simulink model "multi_kanal_V2"  (R2024a)
settings: Solver=VariableStepAuto  StartTime=0.0  StopTime=1000  RelTol=1e-9  AbsTol=1e-10
libraries: simulink x13, matrix_library x3, sharedutil x2, aerolibutil x1
settings Model: Creator=evgenijkondratev  LastModifiedBy=evgenijkondratev

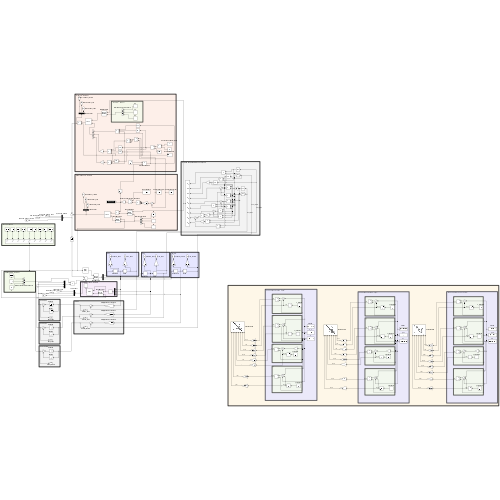
[thumbnail: Simulink's stored preview of the top-level diagram]
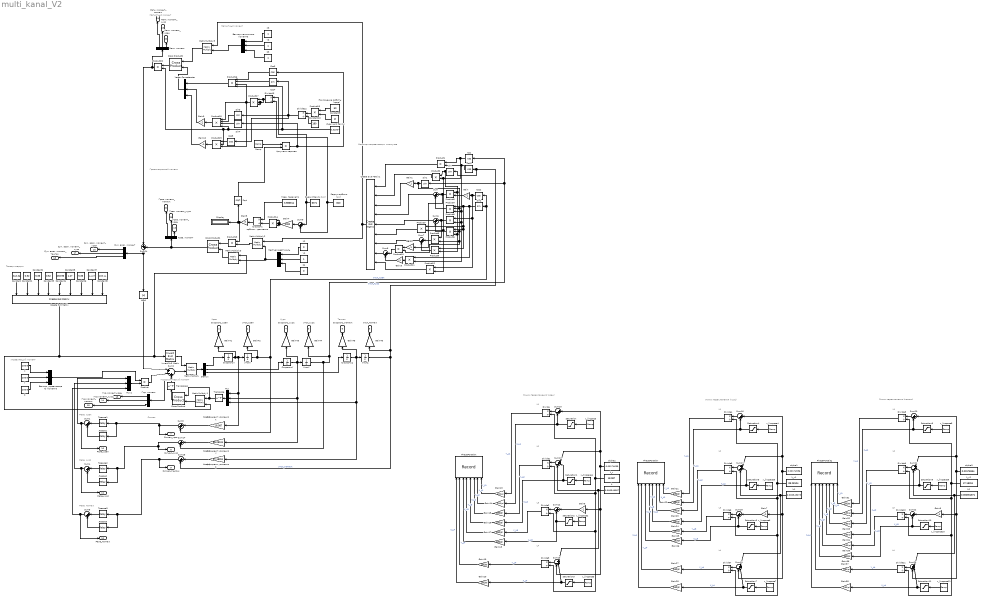
== system multi_kanal_V2 ==
  note: L3
  note: L4
  note: Крен
  note: Магнитный момент
  note: Линии переключения (крен)
  note: L4
  note: Линии переключения (курс)
  note: Линии переключения (тангаж)
  note: L3
  note: L1
  note: Реле, тангаж
  note: L2
  note: L4
  note: L1
  note: L1
  note: L3
  note: Сигнал
  note: Матрица направляющих косинусов
  note: Тензор инерции
  note: L2
  note: Реле, курс
  note: L2
  note: Управляющий момент
  note: Курс
  note: Тангаж
  note: Реле, крен
  note: Гироскопический момент
  note: Гравитационный момент
  note: Магнитный момент
  Abs1 : Abs  SaturateOnIntegerOverflow=off
  Constant : Constant  Value=363.86
  Constant1 : Constant  Value=0.52
  Constant10 : Constant  Value=180
  Constant2 : Constant  Value=5.36
  Constant3 : Constant  Value=0.52
  Constant4 : Constant  Value=233.96
  Constant5 : Constant  Value=1.27
  Constant6 : Constant  Value=5.36
  Constant7 : Constant  Value=14.27
  Constant8 : Constant  Value=285.14
  Constant9 : Constant  Value=pi
  Cos{,1..3,5} (5 alike) : Trigonometry  Operator=cos
  Cos4 : Trigonometry
  Create 3x3 Matrix : sharedutil/Create 3x3 Matrix  aMode=aMode
      settings: LibrarySourceBlock=aerolibutil/Create 3x3 Matrix
  Create 3x3 Matrix1 : sharedutil/Create 3x3 Matrix  aMode=aMode
      settings: LibrarySourceBlock=aerolibutil/Create 3x3 Matrix
  Cross Product : matrix_library/Cross Product
  Cross Product1 : matrix_library/Cross Product
  Cross Product2 : matrix_library/Cross Product
  Demux : Demux  Outputs=3
  Display : Display
  Divide{,1..13} (14 alike) : Product  Inputs=*/
  Gain{,1..3,6..8,10} (8 alike) : Gain  Gain=-1
  Gain{13..28,31..38,41..46} (30 alike) : Gain  Gain=180/pi
  Gain4 : Gain  Gain=1000
  Gain5 : Gain  Gain=3
  Gain9 : Gain  Gain=-2
  Invert 3x3 Matrix : aerolibutil/Invert  3x3 Matrix
  MatrixMultiply{,1..3,5} (5 alike) : Product  Multiplication=Matrix(*)
  Mux : Mux  Inputs=3
  Mux1 : Mux  Inputs=3
  PhasePortraitX : Record  FileSettingsInternal="{\"entries\":[{\"content\":{\"excelSettings\":{\"content\":{},\"type\":\"Streamout.ExcelSettings\"}},\"type\":\"Streamout.FileSettingStorage\",\"uuid\":\"\"}],\"packageUris\":[\"http:\\/\\/schema.mathworks.com\\/mf0\\/streamout_blocks\\/R2020a\"],\"version\":\"1.0\"}"  Layout=[1 1]  SignalsInternal="{\"entries\":[{\"content\":{\"signals\":[{\"content\":{\"blockPath\":[],\"dimensions\":[1],\"domain\":\"\",\"lineColor\":\"#7e2f8e\",\"lineWidth\":2,\"port\":1,\"sid\":[\"\"],\"signalID\":1,\"signalName\":\"X_L4\"},\"type\":\"RecordBlkView.Signal\",\"uuid\":\"\"},{\"content\":{\"blockPath\":[],\"dimensions\":[1],\"domain\":\"\",\"lineColor\":\"#77ac30\",\"lineWidth\":2,\"port\":2,\"sid\":[\"\"],\"signalID\":2,\"signalName\":\"Y_L4\"},\"type\":\"RecordBlkView.Signal\",\"uuid\":\"\"},{\"content\":{\"blockPath\":[],\"dimensions\":[1],\"domain\":\"\",\"lineColor\":\"#4dbeee\",\"lineWidth\":2,\"port\":3,\"sid\":[\"\"],\"signalID\":3,\"signalName\":\"X_L3\"},\"type\":\"RecordBlkView.Signal\",\"uuid\":\"\"},{\"content\":{\"blockPath\":[],\"dimensions\":[1],\"domain\":\"\",\"lineColor\":\"#a2142f\",\"lineWidth\":2,\"port\":4,\"sid\":[\"\"],\"signalID\":4,\"signalName\":\"Y_L3\"},\"type\":\"RecordBlkView.Signal\",\"uuid\":\"\"},{\"content\":{\"blockPath\":[],\"dimensions\":[1],\"domain\":\"\",\"lineColor\":\"#139fff\",\"lineWidth\":2,\"port\":5,\"sid\":[\"\"],\"signalID\":5,\"signalName\":\"X_L2\"},\"type\":\"RecordBlkView.Signal\",\"uuid\":\"\"},{\"content\":{\"blockPath\":[],\"dimensions\":[1],\"domain\":\"\",\"lineColor\":\"#ff6929\",\"lineWidth\":2,\"port\":6,\"sid\":[\"\"],\"signalID\":6,\"signalName\":\"Y_L2\"},\"type\":\"RecordBlkView.Signal\",\"uuid\":\"\"},{\"content\":{\"blockPath\":[],\"dimensions\":[1],\"domain\":\"\",\"lineColor\":\"#b746ff\",\"lineWidth\":2,\"port\":7,\"sid\":[\"\"],\"signalID\":7,\"signalName\":\"X_L1\"},\"type\":\"RecordBlkView.Signal\",\"uuid\":\"\"},{\"content\":{\"blockPath\":[],\"dimensions\":[1],\"domain\":\"\",\"lineColor\":\"#64d413\",\"lineWidth\":2,\"port\":8,\"sid\":[\"\"],\"signalID\":8,\"signalName\":\"Y_L1\"},\"type\":\"RecordBlkView.Signal\",\"uuid\":\"\"}]},\"type\":\"RecordBlkView.InputSignals\",\"uuid\":\"\"}],\"packageUris\":[\"http:\\/\\/schema.mathworks.com\\/mf0\\/streamout_blocks\\/R2020a\"],\"version\":\"1.0\"}"  VisualizationBindings="{\"xyplotplugin\":{\"info\":[{\"series\":[],\"subplotID\":1}]}}"  CompatibilityTag=XY
  PhasePortraitY : Record  FileSettingsInternal="{\"entries\":[{\"content\":{\"excelSettings\":{\"content\":{},\"type\":\"Streamout.ExcelSettings\"}},\"type\":\"Streamout.FileSettingStorage\",\"uuid\":\"\"}],\"packageUris\":[\"http:\\/\\/schema.mathworks.com\\/mf0\\/streamout_blocks\\/R2020a\"],\"version\":\"1.0\"}"  Layout=[1 1]  SignalsInternal="{\"entries\":[{\"content\":{\"signals\":[{\"content\":{\"blockPath\":[],\"dimensions\":[1],\"domain\":\"\",\"lineColor\":\"#4dbeee\",\"lineWidth\":2,\"port\":1,\"sid\":[\"\"],\"signalID\":1,\"signalName\":\"X_L4\"},\"type\":\"RecordBlkView.Signal\",\"uuid\":\"\"},{\"content\":{\"blockPath\":[],\"dimensions\":[1],\"domain\":\"\",\"lineColor\":\"#a2142f\",\"lineWidth\":2,\"port\":2,\"sid\":[\"\"],\"signalID\":2,\"signalName\":\"Y_L4\"},\"type\":\"RecordBlkView.Signal\",\"uuid\":\"\"},{\"content\":{\"blockPath\":[],\"dimensions\":[1],\"domain\":\"\",\"lineColor\":\"#139fff\",\"lineWidth\":2,\"port\":3,\"sid\":[\"\"],\"signalID\":3,\"signalName\":\"X_L3\"},\"type\":\"RecordBlkView.Signal\",\"uuid\":\"\"},{\"content\":{\"blockPath\":[],\"dimensions\":[1],\"domain\":\"\",\"lineColor\":\"#ff6929\",\"lineWidth\":2,\"port\":4,\"sid\":[\"\"],\"signalID\":4,\"signalName\":\"Y_L3\"},\"type\":\"RecordBlkView.Signal\",\"uuid\":\"\"},{\"content\":{\"blockPath\":[],\"dimensions\":[1],\"domain\":\"\",\"lineColor\":\"#b746ff\",\"lineWidth\":2,\"port\":5,\"sid\":[\"\"],\"signalID\":5,\"signalName\":\"X_L2\"},\"type\":\"RecordBlkView.Signal\",\"uuid\":\"\"},{\"content\":{\"blockPath\":[],\"dimensions\":[1],\"domain\":\"\",\"lineColor\":\"#64d413\",\"lineWidth\":2,\"port\":6,\"sid\":[\"\"],\"signalID\":6,\"signalName\":\"Y_L2\"},\"type\":\"RecordBlkView.Signal\",\"uuid\":\"\"},{\"content\":{\"blockPath\":[],\"dimensions\":[1],\"domain\":\"\",\"lineColor\":\"#ff13a6\",\"lineWidth\":2,\"port\":7,\"sid\":[\"\"],\"signalID\":7,\"signalName\":\"X_L1\"},\"type\":\"RecordBlkView.Signal\",\"uuid\":\"\"},{\"content\":{\"blockPath\":[],\"dimensions\":[1],\"domain\":\"\",\"lineColor\":\"#fe330a\",\"lineWidth\":2,\"port\":8,\"sid\":[\"\"],\"signalID\":8,\"signalName\":\"Y_L1\"},\"type\":\"RecordBlkView.Signal\",\"uuid\":\"\"}]},\"type\":\"RecordBlkView.InputSignals\",\"uuid\":\"\"}],\"packageUris\":[\"http:\\/\\/schema.mathworks.com\\/mf0\\/streamout_blocks\\/R2020a\"],\"version\":\"1.0\"}"  VisualizationBindings="{\"xyplotplugin\":{\"info\":[{\"series\":[],\"subplotID\":1}]}}"  CompatibilityTag=XY
  PhasePortraitZ : Record  FileSettingsInternal="{\"entries\":[{\"content\":{\"excelSettings\":{\"content\":{},\"type\":\"Streamout.ExcelSettings\"}},\"type\":\"Streamout.FileSettingStorage\",\"uuid\":\"\"}],\"packageUris\":[\"http:\\/\\/schema.mathworks.com\\/mf0\\/streamout_blocks\\/R2020a\"],\"version\":\"1.0\"}"  Layout=[1 1]  SignalsInternal="{\"entries\":[{\"content\":{\"signals\":[{\"content\":{\"blockPath\":[],\"dimensions\":[1],\"domain\":\"\",\"lineColor\":\"#22b573\",\"lineWidth\":2,\"plots\":[ 1 ],\"port\":1,\"sid\":[\"\"],\"signalID\":1,\"signalName\":\"X_L4\"},\"type\":\"RecordBlkView.Signal\",\"uuid\":\"\"},{\"content\":{\"blockPath\":[],\"dimensions\":[1],\"domain\":\"\",\"lineColor\":\"#7e2f8e\",\"lineWidth\":2,\"plots\":[ 1 ],\"port\":2,\"sid\":[\"\"],\"signalID\":2,\"signalName\":\"Y_L4\"},\"type\":\"RecordBlkView.Signal\",\"uuid\":\"\"},{\"content\":{\"blockPath\":[],\"dimensions\":[1],\"domain\":\"\",\"lineColor\":\"#fe330a\",\"lineWidth\":2,\"port\":3,\"sid\":[\"\"],\"signalID\":3,\"signalName\":\"X_L3\"},\"type\":\"RecordBlkView.Signal\",\"uuid\":\"\"},{\"content\":{\"blockPath\":[],\"dimensions\":[1],\"domain\":\"\",\"lineColor\":\"#22b573\",\"lineWidth\":2,\"port\":4,\"sid\":[\"\"],\"signalID\":4,\"signalName\":\"Y_L3\"},\"type\":\"RecordBlkView.Signal\",\"uuid\":\"\"},{\"content\":{\"blockPath\":[],\"dimensions\":[1],\"domain\":\"\",\"lineColor\":\"#0072bd\",\"lineWidth\":2,\"port\":5,\"sid\":[\"\"],\"signalID\":5,\"signalName\":\"X_L2\"},\"type\":\"RecordBlkView.Signal\",\"uuid\":\"\"},{\"content\":{\"blockPath\":[],\"dimensions\":[1],\"domain\":\"\",\"lineColor\":\"#64d413\",\"lineWidth\":2,\"port\":6,\"sid\":[\"\"],\"signalID\":6,\"signalName\":\"Y_L2\"},\"type\":\"RecordBlkView.Signal\",\"uuid\":\"\"},{\"content\":{\"blockPath\":[],\"dimensions\":[1],\"domain\":\"\",\"lineColor\":\"#edb120\",\"lineWidth\":2,\"port\":7,\"sid\":[\"\"],\"signalID\":7,\"signalName\":\"X_L1\"},\"type\":\"RecordBlkView.Signal\",\"uuid\":\"\"},{\"content\":{\"blockPath\":[],\"dimensions\":[1],\"domain\":\"\",\"lineColor\":\"#7e2f8e\",\"lineWidth\":2,\"port\":8,\"sid\":[\"\"],\"signalID\":8,\"signalName\":\"Y_L1\"},\"type\":\"RecordBlkView.Signal\",\"uuid\":\"\"}]},\"type\":\"RecordBlkView.InputSignals\",\"uuid\":\"\"}],\"packageUris\":[\"http:\\/\\/schema.mathworks.com\\/mf0\\/streamout_blocks\\/R2020a\"],\"version\":\"1.0\"}"  VisualizationBindings="{\"xyplotplugin\":{\"info\":[{\"series\":[{\"bindingParametersList\":[{\"parameter\":\"X-Axis\",\"signalID\":1,\"signalName\":\"X_L4\"},{\"parameter\":\"Y-Axis\",\"signalID\":2,\"signalName\":\"Y_L4\"}],\"seriesID\":0}],\"subplotID\":1}]}}"  CompatibilityTag=XY
  Product{,1..3,5,7..13,15,20} (14 alike) : Product
  Product{4,6,14,17,19} (5 alike) : Product  Inputs=3
  Product16 : Product  Inputs=4
  Product18 : Product  Inputs=4
  Ramp : simulink/Sources/Ramp  slope=1  start=0  InitialOutput=0
  Saturation{,1..11} (12 alike) : Saturate  UpperLimit=0.15  LowerLimit=-0.15
  Sin{,1..4} (5 alike) : Trigonometry
  Sqrt : Sqrt
  Sum{,1,3..9,14..15,24} (12 alike) : Sum  Inputs=|++
  Sum{10,12,16,18,20,22} (6 alike) : Sum  Inputs=|+-
  Sum{11,13,17,19,21,23} (6 alike) : Sum  Inputs=|+--
  Sum2 : Sum  Inputs=|+-+
  Transpose : Math  Operator=transpose
  Transpose1 : Math  Operator=transpose
  Vector Concatenate : Concatenate  NumInputs=3
  X : Constant  Value=20e-3
  X2 : Constant  Value=0
  X3 : Constant
  Y : Constant  Value=20e-3
  Y2 : Constant
  Y3 : Constant
  Z : Constant  Value=20e-3
  Z2 : Constant  Value=0
  Z3 : Constant
  alpha1 : Constant  Value=0.00174536
  alpha2 : Constant  Value=0.00174639
  alpha3 : Constant  Value=0.00175934
  h : Constant  Value=0.000349087
  h1 : Constant  Value=0.000349073
  h2 : Constant  Value=0.000351871
  k_x : Constant  Value=18.087
  k_x1 : Constant  Value=89.28104
  k_x2 : Constant  Value=37.18251
  x_linspace{,1..11} (12 alike) : simulink/Sources/Ramp  slope=1  start=0  InitialOutput=-1
  Аргумент перигея : Product
  Вектор магнитного момента : Concatenate  NumInputs=3
  Вектор управляющего момента : Concatenate  NumInputs=3
  Гир. момент : Demux  Outputs=3
  Грав. момент : Demux  Outputs=3
  Грав. параметр : Constant  Value=3.986e14
  Индукция Земли : Constant  Value=0.315e-4
  Коэффициент усиления X : Gain  Gain=18.087
  Коэффициент усиления Y : Gain  Gain=89.28104
  Коэффициент усиления Z : Gain  Gain=37.18251
  Левое1 : Relay  OnSwitchValue=-0.00174639+0.000349087  OffSwitchValue=-0.00174639  OnOutputValue=0  OffOutputValue=-1
  Левое2 : Relay  OnSwitchValue=-0.00174536+0.000349073  OffSwitchValue=-0.00174536  OnOutputValue=0  OffOutputValue=-1
  Левое3 : Relay  OnSwitchValue=-0.00175934+0.000351871  OffSwitchValue=-0.00175934  OnOutputValue=0  OffOutputValue=-1
  Магн. момент : Demux  Outputs=3
  Местная вертикаль : Concatenate  NumInputs=3
  Наклонение орбиты (град) : Constant  Value=50
  Правое1 : Relay  OnSwitchValue=0.00174639  OffSwitchValue=0.00174639-0.000349087
  Правое2 : Relay  OnSwitchValue=0.00174536  OffSwitchValue=0.00174536-0.000349073
  Правое3 : Relay  OnSwitchValue=0.00175934  OffSwitchValue=0.00175934-0.000351871
  Радиус Земли (км) : Constant  Value=6371
  Радиус орбиты (км) : Constant  Value=820
  Скорость орбитального движения : Product  Inputs=*/
  СкоростьX : Integrator  InitialCondition=0.00053*pi/180
  СкоростьY : Integrator  InitialCondition=0.00008*pi/180
  СкоростьZ : Integrator  InitialCondition=0.00028*pi/180
  Сум. возм. момент : Demux  Outputs=3
  УголX : Integrator
  УголY : Integrator
  УголZ : Integrator
  Угол_крен : Outport
  Скорость_крен : Outport  Port=2
  Угол_курс : Outport  Port=3
  Скорость_курс : Outport  Port=4
  Угол_тангаж : Outport  Port=5
  Скорость_тангаж : Outport  Port=6
  Сигнал_крен : Outport  Port=7
  Сигнал_курс : Outport  Port=8
  Сигнал_тангаж : Outport  Port=9
  Реле_крен : Outport  Port=10
  Реле_курс : Outport  Port=11
  Реле_тангаж : Outport  Port=12
  Гир.момент_крен : Outport  Port=13
  Гир.момент_курс : Outport  Port=14
  Гир.момент_тангаж : Outport  Port=15
  Сум. возм. момент_крен : Outport  Port=16
  Сум. возм. момент_курс : Outport  Port=17
  Сум. возм. момент_тангаж : Outport  Port=18
  Грав. момент_крен : Outport  Port=19
  Грав. момент_курс : Outport  Port=20
  Грав. момент_тангаж : Outport  Port=21
  Магн. момент_крен : Outport  Port=22
  Магн. момент_курс : Outport  Port=23
  Магн. момент_тангаж : Outport  Port=24
  wires:
  Y2/1 -> Местная вертикаль/2
  Sum17/1 -> Divide5/1
  Ramp/1 -> Аргумент перигея/1
  Z/1 -> Вектор управляющего момента/3
  Cross Product/1 -> Transpose1/1
  x_linspace4/1 -> Saturation4/1
  Divide7/1 -> Gain27/1  "Y_L4"
  Sum15/1 -> Сигнал_тангаж/1, Левое3/1, Правое3/1
  Cos1/1 -> Product1/2, Product11/2, Product5/2, Product4/3
  Product8/1 -> Sum7/1
  Divide9/1 -> Gain33/1  "Y_L2"
  Sum23/1 -> Divide11/1
  Saturation9/1 -> Gain34/1, Sum21/2  "X_L2"
  Z3/1 -> Вектор магнитного момента/3
  Sum21/1 -> Divide9/1
  Mux1/1 -> Product/2
  x_linspace8/1 -> Saturation8/1
  Sum22/1 -> Divide10/1
  Invert 3x3 Matrix/1 -> MatrixMultiply/1
  Saturation/1 -> Gain14/1, Sum10/2  "X_L1"
  Gain25/1 -> PhasePortraitY/4  "Y_L3"
  Demux/2 -> СкоростьY/1
  Gain36/1 -> PhasePortraitZ/3  "X_L3"
  Gain32/1 -> PhasePortraitZ/7  "X_L1"
  Divide6/1 -> Gain25/1  "Y_L3"
  Правое3/1 -> Sum5/1
  k_x1/1 -> Divide7/2, Divide6/2, Divide5/2, Divide4/2
  Saturation6/1 -> Gain26/1, Sum18/2  "X_L3"
  Sum13/1 -> Divide3/1
  Demux/3 -> СкоростьZ/1
  Product15/1 -> Divide12/1
  Product9/1 -> Sum7/2
  Sum7/1 -> Create 3x3 Matrix1/7
  k_x2/1 -> Divide11/2, Divide10/2, Divide9/2, Divide8/2
  Gain28/1 -> PhasePortraitY/1  "X_L4"
  Product1/1 -> Create 3x3 Matrix1/1
  Transpose/1 -> Cross Product/1, MatrixMultiply1/1
  Saturation11/1 -> Gain38/1, Sum23/2  "X_L4"
  Z2/1 -> Местная вертикаль/3
  Divide11/1 -> Gain37/1  "Y_L4"
  Saturation8/1 -> Gain32/1, Sum20/2  "X_L1"
  Gain17/1 -> PhasePortraitX/4  "Y_L3"
  Gain/1 -> Product3/2
  Divide4/1 -> Gain21/1  "Y_L1"
  alpha1/1 -> Gain7/1, Sum19/3, Sum17/1, Sum16/1
  Gain6/1 -> Sum12/1
  Saturation5/1 -> Gain24/1, Sum17/2  "X_L2"
  Gain31/1 -> PhasePortraitZ/8  "Y_L1"
  Gain34/1 -> PhasePortraitZ/5  "X_L2"
  Sum14/1 -> Сигнал_курс/1, Левое2/1, Правое2/1
  h2/1 -> Sum21/3, Sum23/1
  Y3/1 -> Вектор магнитного момента/2
  Create 3x3 Matrix1/1 -> MatrixMultiply2/1, MatrixMultiply5/1
  Sum12/1 -> Divide2/1
  Constant6/1 -> Create 3x3 Matrix/7
  Gain3/1 -> Sum8/2
  Divide2/1 -> Gain17/1  "Y_L3"
  x_linspace3/1 -> Saturation3/1
  Gain19/1 -> PhasePortraitX/2  "Y_L4"
  Gain21/1 -> PhasePortraitY/8  "Y_L1"
  Gain18/1 -> PhasePortraitX/3  "X_L3"
  Divide12/1 -> Sin3/1, Cos4/1, Cos5/1
  Constant4/1 -> Create 3x3 Matrix/5
  Constant7/1 -> Create 3x3 Matrix/8
  Gain2/1 -> Product10/1
  Saturation4/1 -> Gain22/1, Sum16/2  "X_L1"
  X/1 -> Вектор управляющего момента/1
  Constant2/1 -> Create 3x3 Matrix/3
  Местная вертикаль/1 -> MatrixMultiply3/2, MatrixMultiply2/2
  Sum19/1 -> Divide7/1
  Gain27/1 -> PhasePortraitY/2  "Y_L4"
  Gain7/1 -> Sum18/1
  Индукция Земли/1 -> Product20/2, Product19/2, Product18/4, Product16/4
  Левое3/1 -> Sum5/2
  Gain9/1 -> Vector Concatenate/2
  Y/1 -> Вектор управляющего момента/2
  MatrixMultiply2/1 -> Product13/2
  Sin/1 -> Product2/1, Product9/2, Product6/3, Product3/1
  Gain4/1 -> Product14/1, Product14/2, Product14/3
  Divide3/1 -> Gain19/1  "Y_L4"
  h/1 -> Sum11/3, Sum13/1
  Sum9/1 -> Gain4/1
  X2/1 -> Местная вертикаль/1
  Sum16/1 -> Divide4/1
  Constant5/1 -> Create 3x3 Matrix/6
  Gain15/1 -> PhasePortraitX/6  "Y_L2"
  Saturation7/1 -> Gain28/1, Sum19/2  "X_L4"
  Saturation1/1 -> Gain16/1, Sum11/2  "X_L2"
  Sqrt/1 -> Аргумент перигея/2
  Gain5/1 -> Display/1, Sqrt/1, Product13/1
  Cross Product1/1 -> Sum24/2, Грав. момент/1
  Transpose1/1 -> Гир. момент/1, Sum2/3
  Saturation10/1 -> Gain36/1, Sum22/2  "X_L3"
  Product7/1 -> Create 3x3 Matrix1/6
  Constant3/1 -> Create 3x3 Matrix/4
  Sum2/1 -> MatrixMultiply/2
  Product5/1 -> Product8/1, Sum6/1
  Правое1/1 -> Sum1/1
  x_linspace5/1 -> Saturation5/1
  Sum24/1 -> Abs1/1, Сум. возм. момент/1
  Product4/1 -> Sum/2
  Product10/1 -> Sum8/1
  Левое2/1 -> Sum4/2
  Saturation2/1 -> Gain18/1, Sum12/2  "X_L3"
  Product14/1 -> Скорость орбитального движения/2
  Правое2/1 -> Sum4/1
  Sum3/1 -> Сигнал_крен/1, Левое1/1, Правое1/1
  Sum10/1 -> Divide/1
  Sum11/1 -> Divide1/1
  Gain22/1 -> PhasePortraitY/7  "X_L1"
  MatrixMultiply1/1 -> Cross Product/2
  x_linspace9/1 -> Saturation9/1
  Gain1/1 -> Create 3x3 Matrix1/3
  x_linspace10/1 -> Saturation10/1
  Constant10/1 -> Divide12/2
  Радиус орбиты (км)/1 -> Sum9/2, Divide13/2
  Divide10/1 -> Gain35/1  "Y_L3"
  Divide/1 -> Gain13/1  "Y_L1"
  Gain8/1 -> Sum22/1
  x_linspace1/1 -> Saturation1/1
  Коэффициент усиления Y/1 -> Sum14/1
  Грав. параметр/1 -> Скорость орбитального движения/1
  Gain13/1 -> PhasePortraitX/8  "Y_L1"
  Cross Product2/1 -> Product20/1
  Product16/1 -> Vector Concatenate/1
  Gain20/1 -> PhasePortraitX/1  "X_L4"
  Gain16/1 -> PhasePortraitX/5  "X_L2"
  x_linspace/1 -> Saturation/1
  alpha2/1 -> Gain6/1, Sum13/3, Sum11/1, Sum10/1
  Вектор магнитного момента/1 -> MatrixMultiply5/2
  Gain35/1 -> PhasePortraitZ/4  "Y_L3"
  Sin1/1 -> Product10/2, Product8/2, Product6/2, Product4/2, Gain1/1
  Коэффициент усиления Z/1 -> Sum15/1
  Product18/1 -> Gain9/1
  x_linspace11/1 -> Saturation11/1
  Gain33/1 -> PhasePortraitZ/6  "Y_L2"
  Divide13/1 -> Product17/1, Product17/3, Product17/2
  Demux/1 -> СкоростьX/1
  Constant9/1 -> Product15/2
  Вектор управляющего момента/1 -> Product/1
  Product2/1 -> Create 3x3 Matrix1/2
  СкоростьX/1 -> Gain41/1, Mux/1, Коэффициент усиления X/1, УголX/1
  Sum1/1 -> Mux1/1, Реле_крен/1
  Sin2/1 -> Product11/1, Product6/1, Product9/1, Product7/1, Product4/1
  Product12/1 -> Create 3x3 Matrix1/9
  Sum8/1 -> Create 3x3 Matrix1/8
  Product6/1 -> Sum6/2
  Constant1/1 -> Create 3x3 Matrix/2
  Коэффициент усиления X/1 -> Sum3/1
  Sum18/1 -> Divide6/1
  Левое1/1 -> Sum1/2
  k_x/1 -> Divide3/2, Divide2/2, Divide1/2, Divide/2
  Радиус Земли (км)/1 -> Divide13/1, Sum9/1
  X3/1 -> Вектор магнитного момента/1
  Constant/1 -> Create 3x3 Matrix/1
  Divide5/1 -> Gain23/1  "Y_L2"
  Sum/1 -> Create 3x3 Matrix1/4
  Divide8/1 -> Gain31/1  "Y_L1"
  Product3/1 -> Gain2/1, Sum/1
  Constant8/1 -> Create 3x3 Matrix/9
  Cos4/1 -> Product16/2
  Gain37/1 -> PhasePortraitZ/2  "Y_L4"
  Gain14/1 -> PhasePortraitX/7  "X_L1"
  Cos/1 -> Product1/1, Product12/2, Product7/2, Product2/2
  x_linspace6/1 -> Saturation6/1
  Vector Concatenate/1 -> Cross Product2/2
  Sum20/1 -> Divide8/1
  h1/1 -> Sum17/3, Sum19/1
  MatrixMultiply5/1 -> Cross Product2/1
  Gain26/1 -> PhasePortraitY/3  "X_L3"
  Наклонение орбиты (град)/1 -> Product15/1
  MatrixMultiply3/1 -> Cross Product1/2
  Divide1/1 -> Gain15/1  "Y_L2"
  Gain38/1 -> PhasePortraitZ/1  "X_L4"
  Sin3/1 -> Product18/2
  Gain10/1 -> Vector Concatenate/3
  Saturation3/1 -> Gain20/1, Sum13/2  "X_L4"
  x_linspace2/1 -> Saturation2/1
  Cos5/1 -> Product19/1
  Product11/1 -> Gain3/1
  Sin4/1 -> Product18/3
  Product17/1 -> Product19/3, Product18/1, Product16/3
  x_linspace7/1 -> Saturation7/1
  Gain23/1 -> PhasePortraitY/6  "Y_L2"
  Скорость орбитального движения/1 -> Gain5/1
  Gain24/1 -> PhasePortraitY/5  "X_L2"
  Mux/1 -> Transpose/1
  Sum4/1 -> Реле_курс/1, Mux1/2
  Sum5/1 -> Реле_тангаж/1, Mux1/3
  Cos2/1 -> Product12/1, Product5/1, Gain/1
  alpha3/1 -> Gain8/1, Sum23/3, Sum21/1, Sum20/1
  Product13/1 -> Cross Product1/1
  СкоростьY/1 -> Gain43/1, Коэффициент усиления Y/1, Mux/2, УголY/1
  Sum6/1 -> Create 3x3 Matrix1/5
  УголZ/1 -> Gain46/1, Sin/1, Cos1/1, Sum15/2  "Угол_тангаж"
  СкоростьZ/1 -> Gain45/1, УголZ/1, Коэффициент усиления Z/1, Mux/3
  Product/1 -> Sum2/2
  УголY/1 -> Cos/1, Sin1/1, Gain44/1, Sum14/2  "Угол_Курс"
  Product19/1 -> Gain10/1
  Create 3x3 Matrix/1 -> Invert 3x3 Matrix/1, MatrixMultiply3/1, MatrixMultiply1/2
  MatrixMultiply/1 -> Demux/1
  УголX/1 -> Sum3/2, Cos2/1, Sin2/1, Gain42/1  "Угол_крен"
  Аргумент перигея/1 -> Sin4/1, Cos3/1
  Cos3/1 -> Product16/1
  Gain41/1 -> Скорость_крен/1
  Gain42/1 -> Угол_крен/1
  Gain43/1 -> Скорость_курс/1
  Gain44/1 -> Угол_курс/1
  Gain45/1 -> Скорость_тангаж/1
  Gain46/1 -> Угол_тангаж/1
  Гир. момент/1 -> Гир.момент_крен/1
  Гир. момент/2 -> Гир.момент_курс/1
  Гир. момент/3 -> Гир.момент_тангаж/1
  Сум. возм. момент/2 -> Сум. возм. момент_курс/1
  Сум. возм. момент/3 -> Сум. возм. момент_тангаж/1
  Сум. возм. момент/1 -> Сум. возм. момент_крен/1
  Грав. момент/3 -> Грав. момент_крен/1
  Грав. момент/2 -> Грав. момент_курс/1
  Грав. момент/1 -> Грав. момент_тангаж/1
  Product20/1 -> Магн. момент/1, Sum24/1
  Магн. момент/1 -> Магн. момент_тангаж/1
  Магн. момент/3 -> Магн. момент_крен/1
  Магн. момент/2 -> Магн. момент_курс/1
  Abs1/1 -> Sum2/1
